simulink model "TURBINE"  (R2016a)
settings: Solver=VariableStepAuto  StartTime=0.0  StopTime=10.0  RelTol=1e-3
values from neighbouring files (symbols this model uses):
  C_l0 = 1.2195    [zmienne.m]
  COF = 3.0326    [zmienne.m]
  CP_fw = 1.218    [zmienne.m]
  ETA_hp = 0.861    [zmienne.m]
  ETA_lp = 0.861    [zmienne.m]
  G_1t = 1.65    [zmienne.m]
  G_vt = 1.5    [zmienne.m]
  H_4p = 958.4    [zmienne.m]
  H_et = 22.589    [zmienne.m]
  HE_fw2 = 863.76    [zmienne.m]
  I_t = 199642    [zmienne.m]
  J = 5.4027    [Pressurizer_constants.m]    (also in zmienne.m = 5.404)
  K10 = 0.53    [zmienne.m]
  K11 = -0.45    [zmienne.m]
  K12 = 0.1    [zmienne.m]
  K13 = -0.017    [zmienne.m]
  K14 = 0.14    [zmienne.m]
  K15 = 0.85612    [zmienne.m]
  K_1c = 1.27453    [zmienne.m]
  K_1co = 37.74    [zmienne.m]
  K_2c = 1068.8    [zmienne.m]
  K_2co = 32    [zmienne.m]
  K_3co = 1092.8    [zmienne.m]
  K_3t = 431.435    [zmienne.m]
  K_4co = 13    [zmienne.m]
  K_5co = 1054    [zmienne.m]
  K_6co = -18    [zmienne.m]
  K_7co = 0.8833    [zmienne.m]
  K_8co = 0.0166    [zmienne.m]
  K_bhp = 0.1634    [zmienne.m]
  K_blp = 0.2174    [zmienne.m]
  KT_t = 1.414    [zmienne.m]
  ML_co = 41422.9    [zmienne.m]
  N_t0 = 60    [zmienne.m]
  P_co = 1    [zmienne.m]
  P_ct = 790    [zmienne.m]
  P_rt = 160    [zmienne.m]
  PI = 3.141    [zmienne.m]
  tau_1t = 4    [zmienne.m]
  tau_2p = 10    [zmienne.m]
  tau_co = 7    [zmienne.m]
  tau_h1 = 65    [zmienne.m]
  tau_h2 = 22    [zmienne.m]
  tau_r1 = 3    [zmienne.m]
  tau_r2 = 10    [zmienne.m]
  tau_w2 = 2    [zmienne.m]
  tau_w3 = 10    [zmienne.m]
  V_ct = 200    [zmienne.m]
  V_ft = 0.018152    [zmienne.m]
  V_rt = 20000    [zmienne.m]
  W_fw = 1036.39    [zmienne.m]
  W_nt = 9.75    [zmienne.m]
  X10 = 931.8    [zmienne.m]
  X11 = 1180    [zmienne.m]
  X12 = 5.556    [zmienne.m]
  X13 = 402.94    [zmienne.m]
  X9 = 251.31    [zmienne.m]
  Z_t = 0.67    [zmienne.m]
undefined symbols (not defined in the file or in its folder): magnitude
settings Model: Creator=Użytkownik  LastModifiedBy=Użytkownik
settings GRTTargetCC: GeneratePreprocessorConditionals=Use local settings

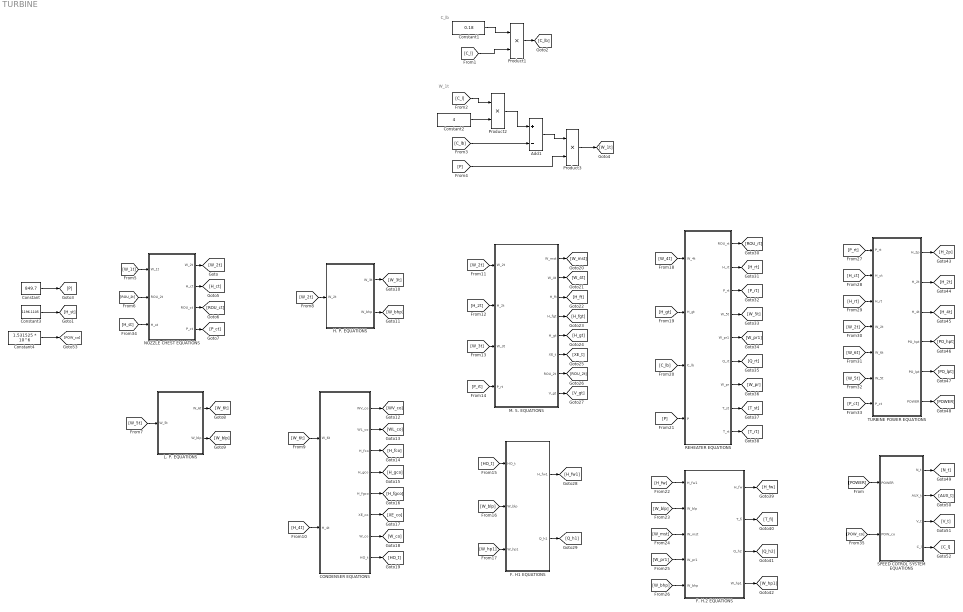
== system TURBINE ==
  note: W_1t
  note: C_lb
  Add1 : Sum  Inputs=+-
  CONDENSER EQUATIONS : Subsystem
  Constant : Constant  Value=849.7
  Constant1 : Constant  Value=0.18
  Constant2 : Constant  Value=4
  Constant3 : Constant  Value=1196.1105
  Constant4 : Constant  Value=1.531525 * 10^6
  "F. H.2 EQUATIONS " : Subsystem
  F. H1 EQUATIONS : Subsystem
  H. P. EQUATIONS : Subsystem
  L. P. EQUATIONS : Subsystem
  M. S. EQUATIONS : Subsystem
  NOZZLE CHEST EQUATIONS : Subsystem
  Product1 : Product
  Product2 : Product
  Product3 : Product
  REHEATER EQUATIONS : Subsystem
  SPEED COTROL SYSTEM EQUATIONS : Subsystem
  TURBINE POWER EQUATIONS : Subsystem
  wires:
  Constant1/1 -> Product1/1
  [C_l] -> Product1/2
  Product1/1 -> [C_lb]
  [C_l] -> Product2/1
  Constant2/1 -> Product2/2
  [C_lb] -> Add1/2
  Product2/1 -> Add1/1
  Add1/1 -> Product3/1
  [P] -> Product3/2
  Product3/1 -> [W_1t]
  NOZZLE CHEST EQUATIONS/1(W_2t) -> [W_2t]
  NOZZLE CHEST EQUATIONS/2(H_ct) -> [H_ct]
  NOZZLE CHEST EQUATIONS/3(ROU_ct) -> [ROU_ct]
  NOZZLE CHEST EQUATIONS/4(P_ct) -> [P_ct]
  L. P. EQUATIONS/1(W_6t) -> [W_6t]
  L. P. EQUATIONS/2(W_blp) -> [W_blp]
  H. P. EQUATIONS/1(W_3t) -> [W_3t]
  H. P. EQUATIONS/2(W_bhp) -> [W_bhp]
  CONDENSER EQUATIONS/1(WV_co) -> [WV_co]
  CONDENSER EQUATIONS/2(WL_co) -> [WL_co]
  CONDENSER EQUATIONS/3(H_fco) -> [H_fco]
  CONDENSER EQUATIONS/4(H_gco) -> [H_gco]
  CONDENSER EQUATIONS/5(H_fgco) -> [H_fgco]
  CONDENSER EQUATIONS/6(XE_co) -> [XE_co]
  CONDENSER EQUATIONS/7(W_co) -> [W_co]
  CONDENSER EQUATIONS/8(HO_t) -> [HO_t]
  M. S. EQUATIONS/1(W_mst) -> [W_mst]
  M. S. EQUATIONS/2(W_4t) -> [W_4t]
  M. S. EQUATIONS/3(H_ft) -> [H_ft]
  M. S. EQUATIONS/4(H_fgt) -> [H_fgt]
  M. S. EQUATIONS/5(H_gt) -> [H_gt]
  M. S. EQUATIONS/6(XE_t) -> [XE_t]
  M. S. EQUATIONS/7(ROU_2t) -> [ROU_2t]
  M. S. EQUATIONS/8(V_gt) -> [V_gt]
  F. H1 EQUATIONS/1(H_fw1) -> [H_fw1]
  F. H1 EQUATIONS/2(Q_h1) -> [Q_h1]
  REHEATER EQUATIONS/1("ROU_rt ") -> [ROU_rt]
  REHEATER EQUATIONS/2(H_rt) -> [H_rt]
  REHEATER EQUATIONS/3(P_rt) -> [P_rt]
  REHEATER EQUATIONS/4(W_5t) -> [W_5t]
  REHEATER EQUATIONS/5(W_pr1) -> [W_pr1]
  REHEATER EQUATIONS/6(Q_rt) -> [Q_rt]
  REHEATER EQUATIONS/7(W_pr) -> [W_pr]
  REHEATER EQUATIONS/8(T_st) -> [T_st]
  REHEATER EQUATIONS/9(T_rt) -> [T_rt]
  "F. H.2 EQUATIONS "/1(H_fw) -> [H_fw]
  "F. H.2 EQUATIONS "/2(T_fi) -> [T_fi]
  "F. H.2 EQUATIONS "/3(Q_h2) -> [Q_h2]
  "F. H.2 EQUATIONS "/4(W_hp1) -> [W_hp1]
  TURBINE POWER EQUATIONS/1(H_2p) -> [H_2p]
  TURBINE POWER EQUATIONS/2(H_2t) -> [H_2t]
  TURBINE POWER EQUATIONS/3(H_4t) -> [H_4t]
  TURBINE POWER EQUATIONS/4(PO_hpt) -> [PO_hpt]
  TURBINE POWER EQUATIONS/5(PO_lpt) -> [PO_lpt]
  TURBINE POWER EQUATIONS/6(POWER) -> [POWER]
  SPEED COTROL SYSTEM EQUATIONS/1(N_t) -> [N_t]
  SPEED COTROL SYSTEM EQUATIONS/2(AUX_t) -> [AUX_t]
  SPEED COTROL SYSTEM EQUATIONS/3(V_t) -> [V_t]
  SPEED COTROL SYSTEM EQUATIONS/4(C_l) -> [C_l]
  [W_1t] -> NOZZLE CHEST EQUATIONS/1(W_1t)
  [ROU_2t] -> NOZZLE CHEST EQUATIONS/2(ROU_2t)
  [W_5t] -> L. P. EQUATIONS/1(W_5t)
  [W_2t] -> H. P. EQUATIONS/1(W_2t)
  [W_6t] -> CONDENSER EQUATIONS/1(W_6t)
  [H_4t] -> CONDENSER EQUATIONS/2(H_4t)
  [W_2t] -> M. S. EQUATIONS/1(W_2t)
  [H_2t] -> M. S. EQUATIONS/2(H_2t)
  [W_3t] -> M. S. EQUATIONS/3(W_3t)
  [P_rt] -> M. S. EQUATIONS/4(P_rt)
  [HO_t] -> F. H1 EQUATIONS/1(HO_t)
  [W_blp] -> F. H1 EQUATIONS/2(W_blp)
  [W_hp1] -> F. H1 EQUATIONS/3(W_hp1)
  [W_4t] -> REHEATER EQUATIONS/1(W_4t)
  [H_gt] -> REHEATER EQUATIONS/2(H_gt)
  [C_lb] -> REHEATER EQUATIONS/3(C_lb)
  [P] -> REHEATER EQUATIONS/4(P)
  [H_fw] -> "F. H.2 EQUATIONS "/1(H_fw1)
  [W_blp] -> "F. H.2 EQUATIONS "/2(W_blp)
  [W_mst] -> "F. H.2 EQUATIONS "/3(W_mst)
  [W_pr1] -> "F. H.2 EQUATIONS "/4(W_pr1)
  [W_bhp] -> "F. H.2 EQUATIONS "/5(W_bhp)
  [P_rt] -> TURBINE POWER EQUATIONS/1(P_rt)
  [H_ct] -> TURBINE POWER EQUATIONS/2(H_ct)
  [H_rt] -> TURBINE POWER EQUATIONS/3(H_rt)
  [W_2t] -> TURBINE POWER EQUATIONS/4(W_2t)
  [W_6t] -> TURBINE POWER EQUATIONS/5(W_6t)
  [W_5t] -> TURBINE POWER EQUATIONS/6(W_5t)
  [P_ct] -> TURBINE POWER EQUATIONS/7(P_ct)
  [POWER] -> SPEED COTROL SYSTEM EQUATIONS/1(POWER)
  Constant/1 -> [P]
  Constant3/1 -> [H_st]
  Constant4/1 -> [POW_co]
  [H_st] -> NOZZLE CHEST EQUATIONS/3(H_st)
  [POW_co] -> SPEED COTROL SYSTEM EQUATIONS/2(POW_co)

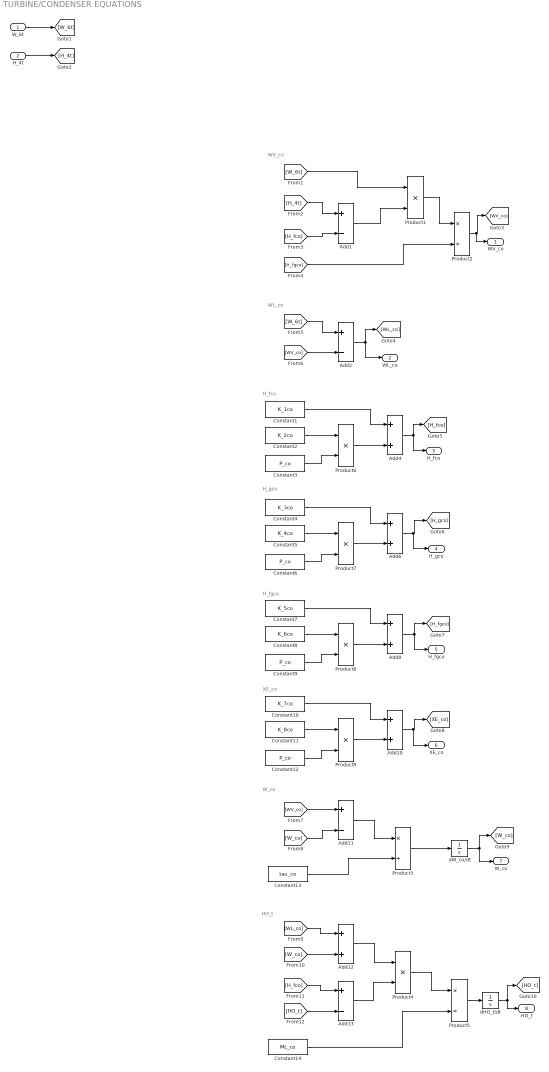
== system TURBINE/CONDENSER EQUATIONS ==
  note: HO_t
  note: W_co
  note: XE_co
  note: H_fgco
  note: H_gco
  note: H_fco
  note: WL_co
  note: WV_co
  W_6t : Inport
  H_4t : Inport  Port=2
  Add{1..2,11,13} (4 alike) : Sum  Inputs=+-
  Add{4,6,8,10,12} (5 alike) : Sum
  Constant1 : Constant  Value=K_1co
  Constant10 : Constant  Value=K_7co
  Constant11 : Constant  Value=K_8co
  Constant{3,6,9,12} (4 alike) : Constant  Value=P_co
  Constant13 : Constant  Value=tau_co
  Constant14 : Constant  Value=ML_co
  Constant2 : Constant  Value=K_2co
  Constant4 : Constant  Value=K_3co
  Constant5 : Constant  Value=K_4co
  Constant7 : Constant  Value=K_5co
  Constant8 : Constant  Value=K_6co
  Product{1,4,6..9} (6 alike) : Product
  Product2 : Product  Inputs=*/
  Product3 : Product  Inputs=*/
  Product5 : Product  Inputs=*/
  dHO_t/dt : Integrator  InitialCondition=69.713
  dW_co/dt : Integrator  InitialCondition=2072.5
  WV_co : Outport
  WL_co : Outport  Port=2
  H_fco : Outport  Port=3
  H_gco : Outport  Port=4
  H_fgco : Outport  Port=5
  XE_co : Outport  Port=6
  W_co : Outport  Port=7
  HO_t : Outport  Port=8
  wires:
  W_6t/1 -> [W_6t]
  H_4t/1 -> [H_4t]
  [H_4t] -> Add1/1
  [H_fco] -> Add1/2
  [W_6t] -> Product1/1
  Add1/1 -> Product1/2
  Product1/1 -> Product2/1
  [H_fgco] -> Product2/2
  Product2/1 -> WV_co/1, [WV_co]
  [W_6t] -> Add2/1
  [WV_co] -> Add2/2
  Add2/1 -> [WL_co], WL_co/1
  Constant2/1 -> Product6/1
  Constant3/1 -> Product6/2
  Constant1/1 -> Add4/1
  Constant5/1 -> Product7/1
  Constant6/1 -> Product7/2
  Constant4/1 -> Add6/1
  Product7/1 -> Add6/2
  Constant8/1 -> Product8/1
  Constant9/1 -> Product8/2
  Constant7/1 -> Add8/1
  Product8/1 -> Add8/2
  Constant11/1 -> Product9/1
  Constant12/1 -> Product9/2
  Constant10/1 -> Add10/1
  Product9/1 -> Add10/2
  Add4/1 -> H_fco/1, [H_fco]
  Add6/1 -> H_gco/1, [H_gco]
  Add8/1 -> [H_fgco], H_fgco/1
  Add10/1 -> XE_co/1, [XE_co]
  [WV_co] -> Add11/1
  [W_co] -> Add11/2
  Add11/1 -> Product3/1
  Constant13/1 -> Product3/2
  Product3/1 -> dW_co/dt/1
  dW_co/dt/1 -> W_co/1, [W_co]
  [W_co] -> Add12/2
  [WL_co] -> Add12/1
  [H_fco] -> Add13/1
  [HO_t] -> Add13/2
  Add12/1 -> Product4/1
  Add13/1 -> Product4/2
  Product4/1 -> Product5/1
  Constant14/1 -> Product5/2
  Product5/1 -> dHO_t/dt/1
  dHO_t/dt/1 -> HO_t/1, [HO_t]
  Product6/1 -> Add4/2

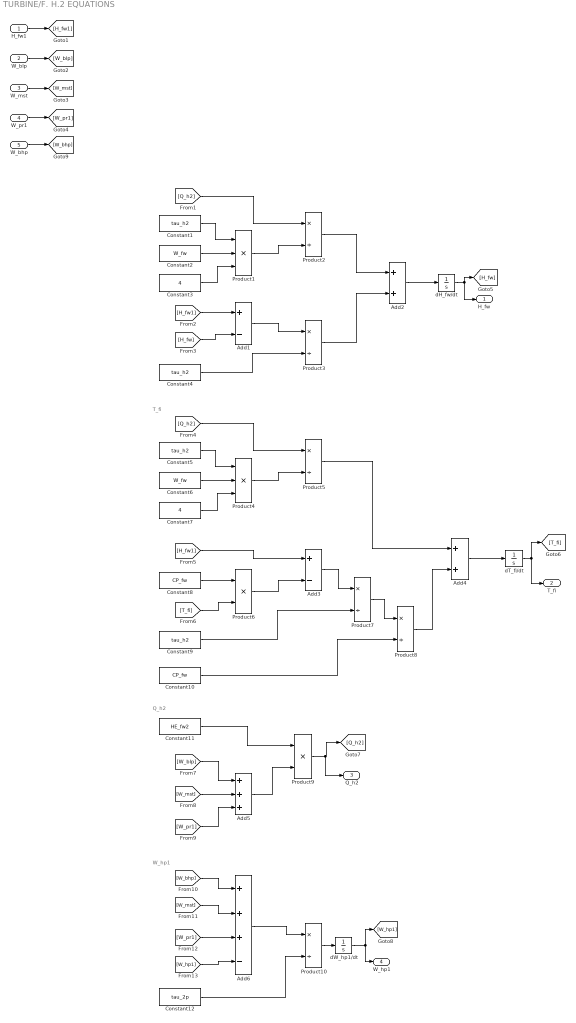
== system TURBINE/F. H.2 EQUATIONS  ==
  note: W_hp1
  note: Q_h2
  note: T_fi
  H_fw1 : Inport
  W_blp : Inport  Port=2
  W_mst : Inport  Port=3
  W_pr1 : Inport  Port=4
  W_bhp : Inport  Port=5
  Add1 : Sum  Inputs=+-
  Add2 : Sum
  Add3 : Sum  Inputs=+-
  Add4 : Sum
  Add5 : Sum  Inputs=3
  Add6 : Sum  Inputs=+++-
  Constant{1,4..5,9} (4 alike) : Constant  Value=tau_h2
  Constant10 : Constant  Value=CP_fw
  Constant11 : Constant  Value=HE_fw2
  Constant12 : Constant  Value=tau_2p
  Constant2 : Constant  Value=W_fw
  Constant3 : Constant  Value=4
  Constant6 : Constant  Value=W_fw
  Constant7 : Constant  Value=4
  Constant8 : Constant  Value=CP_fw
  Product1 : Product  Inputs=3
  Product{2..3,5,7..8,10} (6 alike) : Product  Inputs=*/
  Product4 : Product  Inputs=3
  Product6 : Product
  Product9 : Product
  dH_fw/dt : Integrator  InitialCondition=529.15
  dT_fi/dt : Integrator  InitialCondition=434.3
  dW_hp1/dt : Integrator  InitialCondition=1217.8
  H_fw : Outport
  T_fi : Outport  Port=2
  Q_h2 : Outport  Port=3
  W_hp1 : Outport  Port=4
  wires:
  H_fw1/1 -> [H_fw1]
  W_blp/1 -> [W_blp]
  W_mst/1 -> [W_mst]
  W_pr1/1 -> [W_pr1]
  Constant1/1 -> Product1/1
  Constant2/1 -> Product1/2
  Constant3/1 -> Product1/3
  [Q_h2] -> Product2/1
  Product1/1 -> Product2/2
  [H_fw1] -> Add1/1
  [H_fw] -> Add1/2
  Add1/1 -> Product3/1
  Constant4/1 -> Product3/2
  Product2/1 -> Add2/1
  Product3/1 -> Add2/2
  Add2/1 -> dH_fw/dt/1
  dH_fw/dt/1 -> H_fw/1, [H_fw]
  Constant5/1 -> Product4/1
  Constant6/1 -> Product4/2
  Constant7/1 -> Product4/3
  [Q_h2] -> Product5/1
  Product4/1 -> Product5/2
  Constant8/1 -> Product6/1
  [T_fi] -> Product6/2
  [H_fw1] -> Add3/1
  Product6/1 -> Add3/2
  Add3/1 -> Product7/1
  Constant9/1 -> Product7/2
  Product5/1 -> Add4/1
  [W_blp] -> Add5/1
  [W_mst] -> Add5/2
  [W_pr1] -> Add5/3
  Constant11/1 -> Product9/1
  Add5/1 -> Product9/2
  dT_fi/dt/1 -> T_fi/1, [T_fi]
  Product9/1 -> Q_h2/1, [Q_h2]
  W_bhp/1 -> [W_bhp]
  [W_bhp] -> Add6/1
  [W_mst] -> Add6/2
  [W_pr1] -> Add6/3
  [W_hp1] -> Add6/4
  Add6/1 -> Product10/1
  Constant12/1 -> Product10/2
  Product10/1 -> dW_hp1/dt/1
  dW_hp1/dt/1 -> W_hp1/1, [W_hp1]
  Add4/1 -> dT_fi/dt/1
  Constant10/1 -> Product8/2
  Product7/1 -> Product8/1
  Product8/1 -> Add4/2

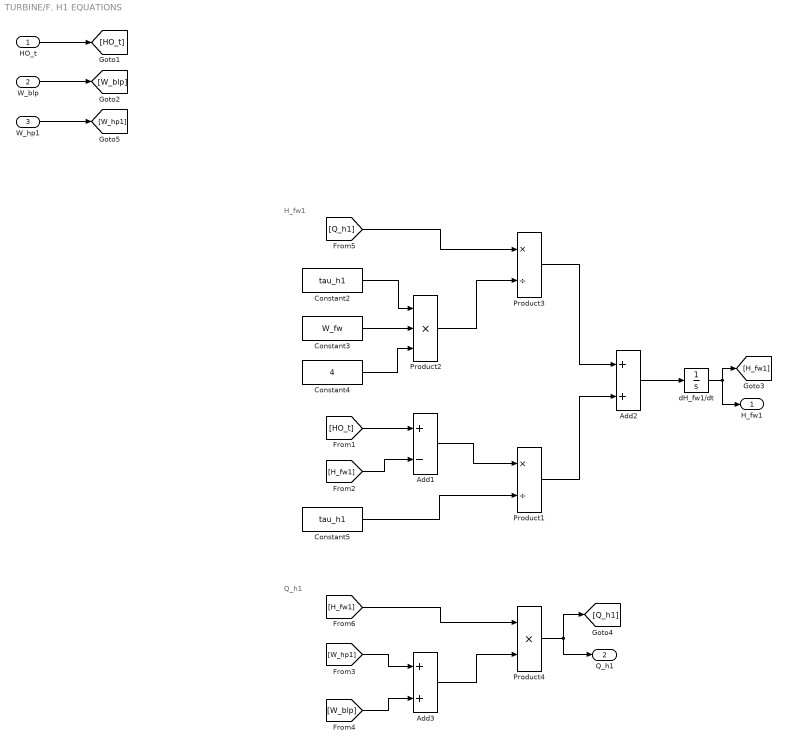
== system TURBINE/F. H1 EQUATIONS ==
  note: Q_h1
  note: H_fw1
  HO_t : Inport
  W_blp : Inport  Port=2
  W_hp1 : Inport  Port=3
  Add1 : Sum  Inputs=+-
  Add2 : Sum
  Add3 : Sum
  Constant2 : Constant  Value=tau_h1
  Constant3 : Constant  Value=W_fw
  Constant4 : Constant  Value=4
  Constant5 : Constant  Value=tau_h1
  Product1 : Product  Inputs=*/
  Product2 : Product  Inputs=***
  Product3 : Product  Inputs=*/
  Product4 : Product
  dH_fw1/dt : Integrator  InitialCondition=280.4
  H_fw1 : Outport
  Q_h1 : Outport  Port=2
  wires:
  HO_t/1 -> [HO_t]
  W_blp/1 -> [W_blp]
  [HO_t] -> Add1/1
  [H_fw1] -> Add1/2
  Add1/1 -> Product1/1
  Constant5/1 -> Product1/2
  Constant2/1 -> Product2/1
  Constant3/1 -> Product2/2
  Constant4/1 -> Product2/3
  Product2/1 -> Product3/2
  [Q_h1] -> Product3/1
  Product3/1 -> Add2/1
  Product1/1 -> Add2/2
  Add2/1 -> dH_fw1/dt/1
  dH_fw1/dt/1 -> [H_fw1], H_fw1/1
  [W_hp1] -> Add3/1
  [W_blp] -> Add3/2
  [H_fw1] -> Product4/1
  Add3/1 -> Product4/2
  Product4/1 -> Q_h1/1, [Q_h1]
  W_hp1/1 -> [W_hp1]

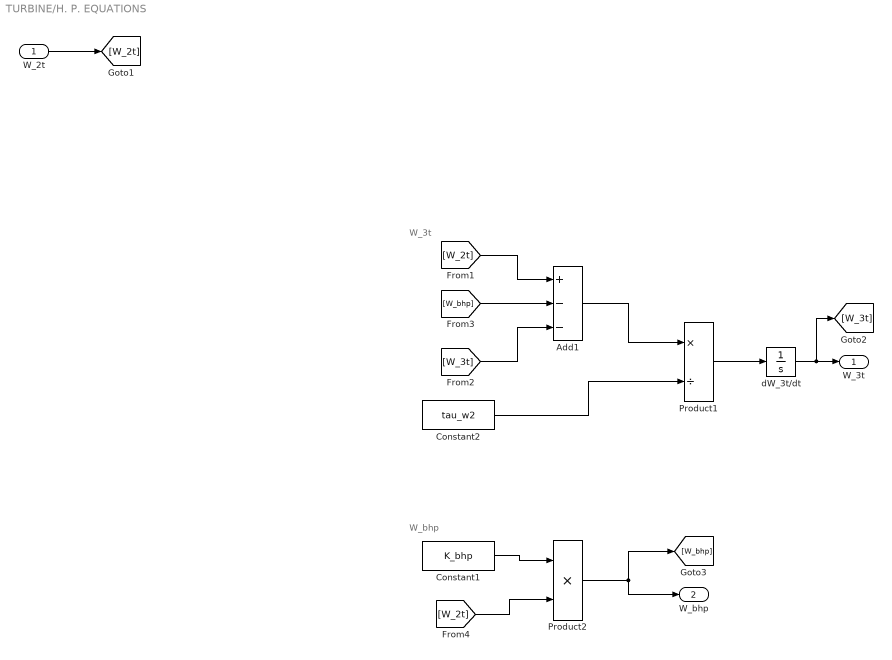
== system TURBINE/H. P. EQUATIONS ==
  note: W_bhp
  note: W_3t
  W_2t : Inport
  Add1 : Sum  Inputs=+--
  Constant1 : Constant  Value=K_bhp
  Constant2 : Constant  Value=tau_w2
  Product1 : Product  Inputs=*/
  Product2 : Product
  dW_3t/dt : Integrator  InitialCondition=3311.56
  W_3t : Outport
  W_bhp : Outport  Port=2
  wires:
  W_2t/1 -> [W_2t]
  [W_2t] -> Add1/1
  [W_bhp] -> Add1/2
  [W_3t] -> Add1/3
  Add1/1 -> Product1/1
  Constant2/1 -> Product1/2
  Product1/1 -> dW_3t/dt/1
  dW_3t/dt/1 -> [W_3t], W_3t/1
  Constant1/1 -> Product2/1
  [W_2t] -> Product2/2
  Product2/1 -> [W_bhp], W_bhp/1

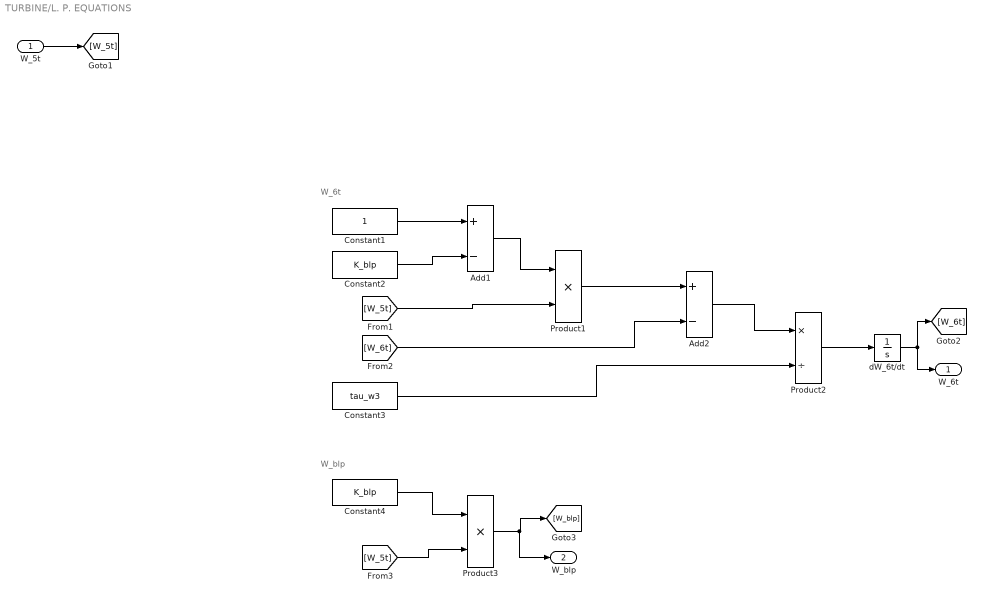
== system TURBINE/L. P. EQUATIONS ==
  note: W_blp
  note: W_6t
  W_5t : Inport
  Add1 : Sum  Inputs=+-
  Add2 : Sum  Inputs=+-
  Constant1 : Constant
  Constant2 : Constant  Value=K_blp
  Constant3 : Constant  Value=tau_w3
  Constant4 : Constant  Value=K_blp
  Product1 : Product
  Product2 : Product  Inputs=*/
  Product3 : Product
  dW_6t/dt : Integrator  InitialCondition=2303
  W_6t : Outport
  W_blp : Outport  Port=2
  wires:
  W_5t/1 -> [W_5t]
  Constant1/1 -> Add1/1
  Constant2/1 -> Add1/2
  Add1/1 -> Product1/1
  [W_5t] -> Product1/2
  Product1/1 -> Add2/1
  [W_6t] -> Add2/2
  Add2/1 -> Product2/1
  Constant3/1 -> Product2/2
  Product2/1 -> dW_6t/dt/1
  dW_6t/dt/1 -> [W_6t], W_6t/1
  Constant4/1 -> Product3/1
  [W_5t] -> Product3/2
  Product3/1 -> W_blp/1, [W_blp]

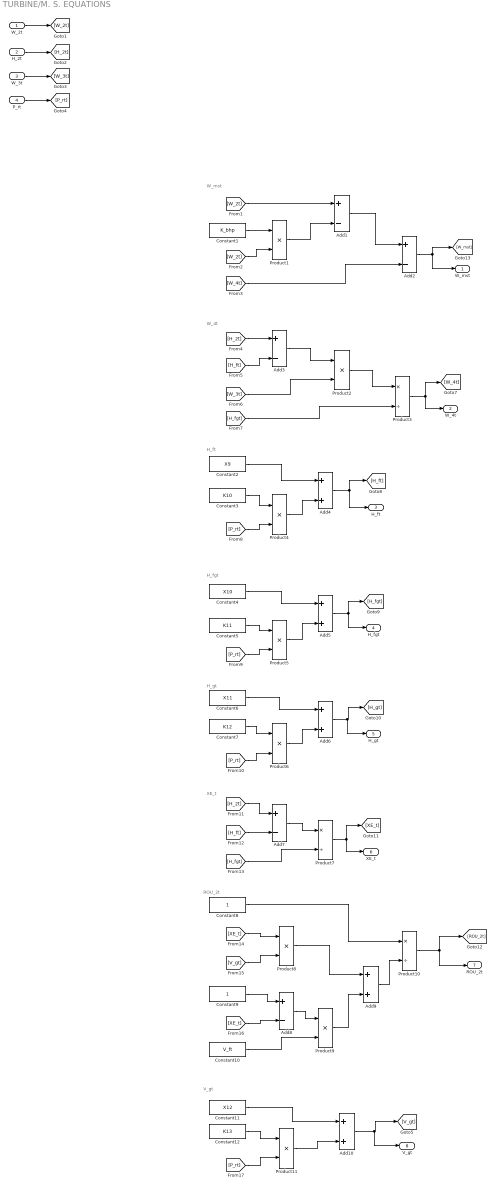
== system TURBINE/M. S. EQUATIONS ==
  note: V_gt
  note: ROU_2t
  note: XE_t
  note: H_gt
  note: H_fgt
  note: H_ft
  note: W_4t
  note: W_mst
  W_2t : Inport
  H_2t : Inport  Port=2
  W_3t : Inport  Port=3
  P_rt : Inport  Port=4
  Add{1..3,7..8} (5 alike) : Sum  Inputs=+-
  Add{4..6,9..10} (5 alike) : Sum
  Constant1 : Constant  Value=K_bhp
  Constant10 : Constant  Value=V_ft
  Constant11 : Constant  Value=X12
  Constant12 : Constant  Value=K13
  Constant2 : Constant  Value=X9
  Constant3 : Constant  Value=K10
  Constant4 : Constant  Value=X10
  Constant5 : Constant  Value=K11
  Constant6 : Constant  Value=X11
  Constant7 : Constant  Value=K12
  Constant8 : Constant
  Constant9 : Constant
  Product{1..2,4..6,8..9,11} (8 alike) : Product
  Product10 : Product  Inputs=*/
  Product3 : Product  Inputs=*/
  Product7 : Product  Inputs=*/
  W_mst : Outport
  W_4t : Outport  Port=2
  H_ft : Outport  Port=3
  H_fgt : Outport  Port=4
  H_gt : Outport  Port=5
  XE_t : Outport  Port=6
  ROU_2t : Outport  Port=7
  V_gt : Outport  Port=8
  wires:
  W_2t/1 -> [W_2t]
  H_2t/1 -> [H_2t]
  W_3t/1 -> [W_3t]
  P_rt/1 -> [P_rt]
  Constant1/1 -> Product1/1
  [W_2t] -> Product1/2
  [W_2t] -> Add1/1
  Product1/1 -> Add1/2
  Add1/1 -> Add2/1
  [W_4t] -> Add2/2
  Add2/1 -> W_mst/1, [W_mst]
  [H_2t] -> Add3/1
  [H_ft] -> Add3/2
  Add3/1 -> Product2/1
  [W_3t] -> Product2/2
  Product2/1 -> Product3/1
  [H_fgt] -> Product3/2
  Product3/1 -> W_4t/1, [W_4t]
  Constant3/1 -> Product4/1
  [P_rt] -> Product4/2
  Constant2/1 -> Add4/1
  Product4/1 -> Add4/2
  Add4/1 -> H_ft/1, [H_ft]
  Constant5/1 -> Product5/1
  [P_rt] -> Product5/2
  Constant4/1 -> Add5/1
  Product5/1 -> Add5/2
  Add5/1 -> H_fgt/1, [H_fgt]
  Constant7/1 -> Product6/1
  [P_rt] -> Product6/2
  Constant6/1 -> Add6/1
  Product6/1 -> Add6/2
  Add6/1 -> H_gt/1, [H_gt]
  [H_2t] -> Add7/1
  [H_ft] -> Add7/2
  Add7/1 -> Product7/1
  [H_fgt] -> Product7/2
  Product7/1 -> XE_t/1, [XE_t]
  [XE_t] -> Product8/1
  [V_gt] -> Product8/2
  Constant9/1 -> Add8/1
  [XE_t] -> Add8/2
  Add8/1 -> Product9/1
  Constant10/1 -> Product9/2
  Product8/1 -> Add9/1
  Product9/1 -> Add9/2
  Constant8/1 -> Product10/1
  Add9/1 -> Product10/2
  Product10/1 -> ROU_2t/1, [ROU_2t]
  Constant12/1 -> Product11/1
  [P_rt] -> Product11/2
  Constant11/1 -> Add10/1
  Product11/1 -> Add10/2
  Add10/1 -> V_gt/1, [V_gt]

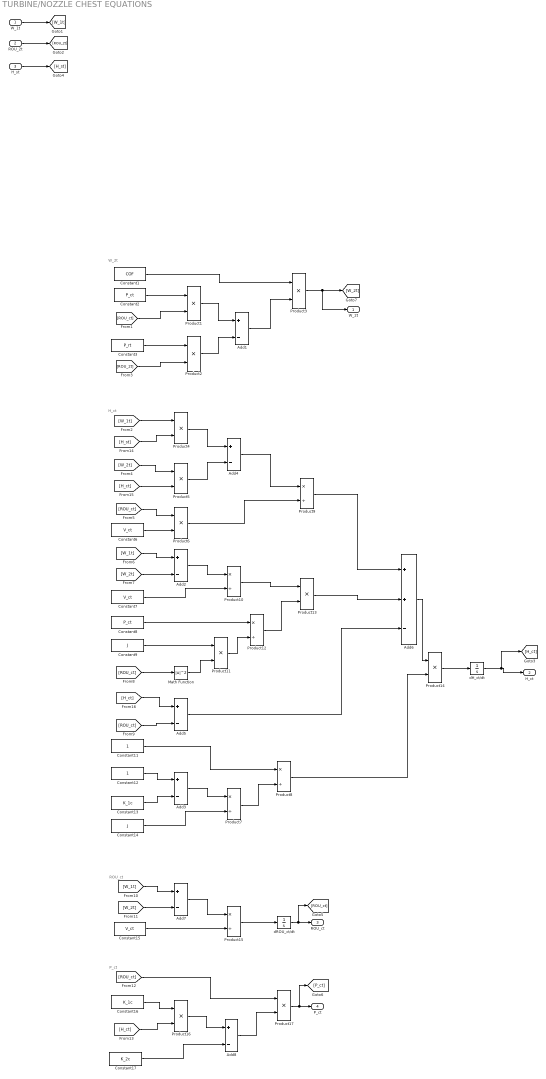
== system TURBINE/NOZZLE CHEST EQUATIONS ==
  note: P_ct
  note: ROU_ct
  note: H_ct
  note: W_2t
  W_1t : Inport
  ROU_2t : Inport  Port=2
  H_st : Inport  Port=3
  Add{1..5,7..8} (7 alike) : Sum  Inputs=+-
  Add6 : Sum  Inputs=++-
  Constant1 : Constant  Value=COF
  Constant11 : Constant
  Constant12 : Constant
  Constant13 : Constant  Value=K_1c
  Constant14 : Constant  Value=J
  Constant15 : Constant  Value=V_ct
  Constant16 : Constant  Value=K_1c
  Constant17 : Constant  Value=K_2c
  Constant2 : Constant  Value=P_ct
  Constant3 : Constant  Value=P_rt
  Constant6 : Constant  Value=V_ct
  Constant7 : Constant  Value=V_ct
  Constant8 : Constant  Value=P_ct
  Constant9 : Constant  Value=J
  Math Function : Math  Operator=magnitude^2  SaturateOnIntegerOverflow=on
  Product{1..6,11,13..14,16..17} (11 alike) : Product
  Product{7..10,12,15} (6 alike) : Product  Inputs=*/
  dH_ct/dt : Integrator  InitialCondition=1196.1
  dROU_ct/dt : Integrator  InitialCondition=1.7337
  W_2t : Outport
  H_ct : Outport  Port=2
  ROU_ct : Outport  Port=3
  P_ct : Outport  Port=4
  wires:
  W_1t/1 -> [W_1t]
  ROU_2t/1 -> [ROU_2t]
  Constant3/1 -> Product2/1
  [ROU_2t] -> Product2/2
  Constant2/1 -> Product1/1
  [ROU_ct] -> Product1/2
  Product1/1 -> Add1/1
  Product2/1 -> Add1/2
  Constant1/1 -> Product3/1
  Add1/1 -> Product3/2
  Product3/1 -> W_2t/1, [W_2t]
  [W_1t] -> Product4/1
  [H_st] -> Product4/2
  [W_2t] -> Product5/1
  [H_ct] -> Product5/2
  [ROU_ct] -> Product6/1
  Constant6/1 -> Product6/2
  [W_1t] -> Add2/1
  [W_2t] -> Add2/2
  [ROU_ct] -> Math Function/1
  Constant12/1 -> Add3/1
  Constant13/1 -> Add3/2
  Add3/1 -> Product7/1
  Constant14/1 -> Product7/2
  Constant11/1 -> Product8/1
  Product7/1 -> Product8/2
  Product4/1 -> Add4/1
  Product5/1 -> Add4/2
  Add4/1 -> Product9/1
  Product6/1 -> Product9/2
  Add2/1 -> Product10/1
  Constant7/1 -> Product10/2
  Constant9/1 -> Product11/1
  Math Function/1 -> Product11/2
  Constant8/1 -> Product12/1
  Product11/1 -> Product12/2
  Product10/1 -> Product13/1
  Product12/1 -> Product13/2
  [H_ct] -> Add5/1
  [ROU_ct] -> Add5/2
  Product9/1 -> Add6/1
  Product13/1 -> Add6/2
  Add5/1 -> Add6/3
  Add6/1 -> Product14/1
  Product8/1 -> Product14/2
  Product14/1 -> dH_ct/dt/1
  dH_ct/dt/1 -> [H_ct], H_ct/1
  [W_2t] -> Add7/2
  [W_1t] -> Add7/1
  Add7/1 -> Product15/1
  Constant15/1 -> Product15/2
  Product15/1 -> dROU_ct/dt/1
  dROU_ct/dt/1 -> [ROU_ct], ROU_ct/1
  Constant16/1 -> Product16/1
  [H_ct] -> Product16/2
  Product16/1 -> Add8/1
  Constant17/1 -> Add8/2
  [ROU_ct] -> Product17/1
  Add8/1 -> Product17/2
  Product17/1 -> [P_ct], P_ct/1
  H_st/1 -> [H_st]

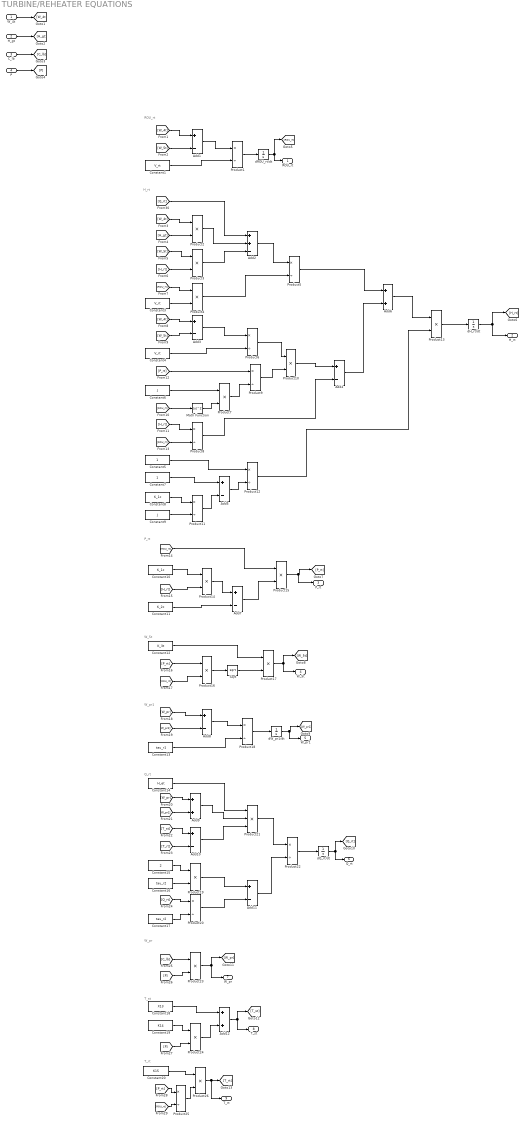
== system TURBINE/REHEATER EQUATIONS ==
  note: T_rt
  note: T_st
  note: W_pr
  note: Q_rt
  note: W_pr1
  note: W_5t
  note: P_rt
  note: H_rt
  note: ROU_rt
  W_4t : Inport
  H_gt : Inport  Port=2
  C_lb : Inport  Port=3
  P : Inport  Port=4
  Add{1,3..5,7..8,10..11} (8 alike) : Sum  Inputs=+-
  Add12 : Sum
  Add2 : Sum  Inputs=++-
  Add6 : Sum
  Add9 : Sum
  Constant1 : Constant  Value=V_rt
  Constant10 : Constant  Value=K_1c
  Constant11 : Constant  Value=K_2c
  Constant12 : Constant  Value=K_3t
  Constant13 : Constant  Value=tau_r1
  Constant14 : Constant  Value=H_et
  Constant15 : Constant  Value=2
  Constant16 : Constant  Value=tau_r2
  Constant17 : Constant  Value=tau_r2
  Constant18 : Constant  Value=X13
  Constant19 : Constant  Value=K14
  Constant20 : Constant  Value=K15
  Constant3 : Constant  Value=V_rt
  Constant4 : Constant  Value=V_rt
  Constant5 : Constant
  Constant6 : Constant  Value=J
  Constant7 : Constant
  Constant8 : Constant  Value=K_1c
  Constant9 : Constant  Value=J
  Math Function : Math  Operator=magnitude^2  SaturateOnIntegerOverflow=on
  Product{1,5..6,8..9,11..12,18,20,22,25} (11 alike) : Product  Inputs=*/
  Product{2..4,7,10,13..17,19,23..24,26} (14 alike) : Product
  Product21 : Product  Inputs=3
  Sqrt : Sqrt  SaturateOnIntegerOverflow=on
  dH_rt/dt : Integrator  InitialCondition=1269.7
  dQ_rt/dt : Integrator  InitialCondition=216931
  dROU_rt/dt : Integrator  InitialCondition=0.291
  dW_pr1/dt : Integrator  InitialCondition=186.36
  "ROU_rt " : Outport
  H_rt : Outport  Port=2
  P_rt : Outport  Port=3
  W_5t : Outport  Port=4
  W_pr1 : Outport  Port=5
  Q_rt : Outport  Port=6
  W_pr : Outport  Port=7
  T_st : Outport  Port=8
  T_rt : Outport  Port=9
  wires:
  W_4t/1 -> [W_4t]
  H_gt/1 -> [H_gt]
  C_lb/1 -> [C_lb]
  P/1 -> [P]
  [W_5t] -> Add1/2
  [W_4t] -> Add1/1
  Add1/1 -> Product1/1
  Constant1/1 -> Product1/2
  Product1/1 -> dROU_rt/dt/1
  dROU_rt/dt/1 -> "ROU_rt "/1, [ROU_rt]
  [H_gt] -> Product2/2
  [W_4t] -> Product2/1
  [H_rt] -> Product3/2
  [W_5t] -> Product3/1
  Constant3/1 -> Product4/2
  [ROU_rt] -> Product4/1
  [Q_rt] -> Add2/1
  Product2/1 -> Add2/2
  Product3/1 -> Add2/3
  Add2/1 -> Product5/1
  Product4/1 -> Product5/2
  [W_4t] -> Add3/1
  [W_5t] -> Add3/2
  Add3/1 -> Product6/1
  Constant4/1 -> Product6/2
  [ROU_rt] -> Math Function/1
  Constant6/1 -> Product7/1
  Math Function/1 -> Product7/2
  [ROU_rt] -> Product8/2
  [H_rt] -> Product8/1
  Product8/1 -> Add4/2
  [P_rt] -> Product9/1
  Product6/1 -> Product10/1
  Constant9/1 -> Product11/2
  Constant8/1 -> Product11/1
  Constant7/1 -> Add5/1
  Product11/1 -> Add5/2
  Constant5/1 -> Product12/1
  Add5/1 -> Product12/2
  Product12/1 -> Product13/2
  Product5/1 -> Add6/1
  dH_rt/dt/1 -> H_rt/1, [H_rt]
  Constant10/1 -> Product14/1
  [H_rt] -> Product14/2
  Product14/1 -> Add7/1
  Constant11/1 -> Add7/2
  [ROU_rt] -> Product15/1
  Add7/1 -> Product15/2
  Product15/1 -> P_rt/1, [P_rt]
  [P_rt] -> Product16/1
  [ROU_rt] -> Product16/2
  Product16/1 -> Sqrt/1
  Constant12/1 -> Product17/1
  Sqrt/1 -> Product17/2
  Product17/1 -> [W_5t], W_5t/1
  [W_pr1] -> Add8/2
  [W_pr] -> Add8/1
  Add8/1 -> Product18/1
  Constant13/1 -> Product18/2
  Product18/1 -> dW_pr1/dt/1
  dW_pr1/dt/1 -> W_pr1/1, [W_pr1]
  [W_pr1] -> Add9/2
  [W_pr] -> Add9/1
  [T_rt] -> Add10/2
  [T_st] -> Add10/1
  Constant16/1 -> Product19/2
  Constant15/1 -> Product19/1
  [Q_rt] -> Product20/1
  Constant17/1 -> Product20/2
  Constant14/1 -> Product21/1
  Add9/1 -> Product21/2
  Add10/1 -> Product21/3
  Product19/1 -> Add11/1
  Product20/1 -> Add11/2
  Product21/1 -> Product22/1
  Add11/1 -> Product22/2
  Product22/1 -> dQ_rt/dt/1
  dQ_rt/dt/1 -> Q_rt/1, [Q_rt]
  [C_lb] -> Product23/1
  [P] -> Product23/2
  Product23/1 -> W_pr/1, [W_pr]
  Constant19/1 -> Product24/1
  [P] -> Product24/2
  Constant18/1 -> Add12/1
  Product24/1 -> Add12/2
  Add12/1 -> T_st/1, [T_st]
  Constant20/1 -> Product26/1
  Product7/1 -> Product9/2
  Add6/1 -> Product13/1
  Product13/1 -> dH_rt/dt/1
  [P_rt] -> Product25/1
  [ROU_rt] -> Product25/2
  Product25/1 -> Product26/2
  Product26/1 -> T_rt/1, [T_rt]
  Product9/1 -> Product10/2
  Product10/1 -> Add4/1
  Add4/1 -> Add6/2

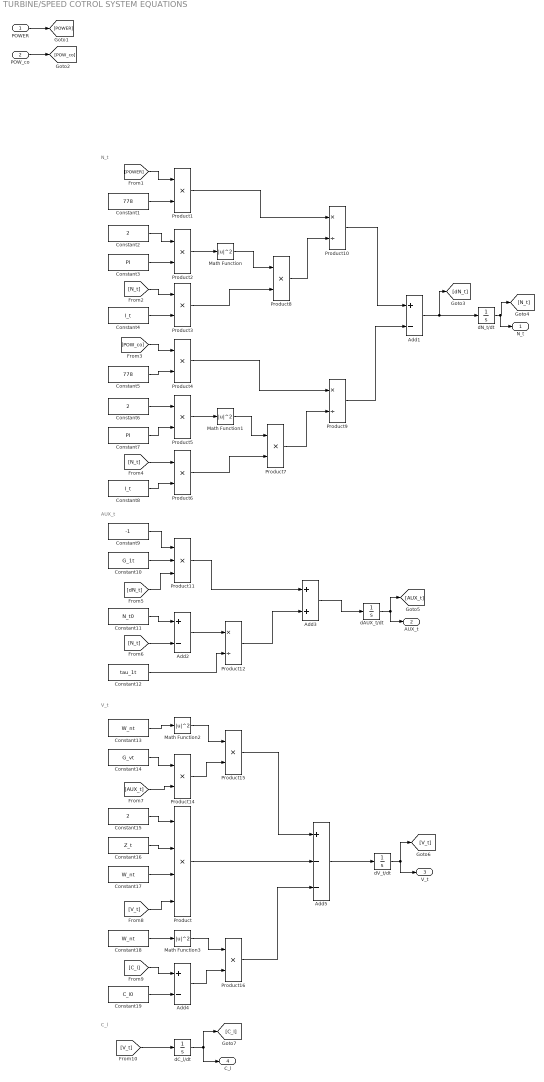
== system TURBINE/SPEED COTROL SYSTEM EQUATIONS ==
  note: C_l
  note: V_t
  note: AUX_t
  note: N_t
  POWER : Inport
  POW_co : Inport  Port=2
  Add1 : Sum  Inputs=+-
  Add2 : Sum  Inputs=+-
  Add3 : Sum
  Add4 : Sum  Inputs=+-
  Add5 : Sum  Inputs=+--
  Constant1 : Constant  Value=778
  Constant10 : Constant  Value=G_1t
  Constant11 : Constant  Value=N_t0
  Constant12 : Constant  Value=tau_1t
  Constant13 : Constant  Value=W_nt
  Constant14 : Constant  Value=G_vt
  Constant15 : Constant  Value=2
  Constant16 : Constant  Value=Z_t
  Constant17 : Constant  Value=W_nt
  Constant18 : Constant  Value=W_nt
  Constant19 : Constant  Value=C_l0
  Constant2 : Constant  Value=2
  Constant3 : Constant  Value=PI
  Constant4 : Constant  Value=I_t
  Constant5 : Constant  Value=778
  Constant6 : Constant  Value=2
  Constant7 : Constant  Value=PI
  Constant8 : Constant  Value=I_t
  Constant9 : Constant  Value=-1
  Math Function{,1..3} (4 alike) : Math  Operator=magnitude^2  SaturateOnIntegerOverflow=on
  Product : Product  Inputs=4
  Product{1..8,14..16} (11 alike) : Product
  Product10 : Product  Inputs=*/
  Product11 : Product  Inputs=3
  Product12 : Product  Inputs=*/
  Product9 : Product  Inputs=*/
  dAUX_t/dt : Integrator
  dC_l/dt : Integrator  InitialCondition=1.2195
  dN_t/dt : Integrator  InitialCondition=60
  dV_t/dt : Integrator
  N_t : Outport
  AUX_t : Outport  Port=2
  V_t : Outport  Port=3
  C_l : Outport  Port=4
  wires:
  POWER/1 -> [POWER]
  POW_co/1 -> [POW_co]
  Constant1/1 -> Product1/2
  [POWER] -> Product1/1
  Constant2/1 -> Product2/1
  Constant3/1 -> Product2/2
  Constant4/1 -> Product3/2
  [N_t] -> Product3/1
  [POW_co] -> Product4/1
  Constant5/1 -> Product4/2
  Constant6/1 -> Product5/1
  Constant7/1 -> Product5/2
  [N_t] -> Product6/1
  Constant8/1 -> Product6/2
  Product2/1 -> Math Function/1
  Product5/1 -> Math Function1/1
  Math Function1/1 -> Product7/1
  Product6/1 -> Product7/2
  Math Function/1 -> Product8/1
  Product3/1 -> Product8/2
  Product4/1 -> Product9/1
  Product7/1 -> Product9/2
  Product8/1 -> Product10/2
  Product1/1 -> Product10/1
  Product10/1 -> Add1/1
  Product9/1 -> Add1/2
  Add1/1 -> [dN_t], dN_t/dt/1
  dN_t/dt/1 -> N_t/1, [N_t]
  Constant9/1 -> Product11/1
  Constant10/1 -> Product11/2
  [dN_t] -> Product11/3
  [N_t] -> Add2/2
  Constant11/1 -> Add2/1
  Product11/1 -> Add3/1
  Constant12/1 -> Product12/2
  dAUX_t/dt/1 -> AUX_t/1, [AUX_t]
  Constant13/1 -> Math Function2/1
  Constant18/1 -> Math Function3/1
  [C_l] -> Add4/1
  Constant19/1 -> Add4/2
  Constant15/1 -> Product/1
  Constant16/1 -> Product/2
  Constant17/1 -> Product/3
  [V_t] -> Product/4
  [AUX_t] -> Product14/2
  Constant14/1 -> Product14/1
  Math Function2/1 -> Product15/1
  Product14/1 -> Product15/2
  Math Function3/1 -> Product16/1
  Add4/1 -> Product16/2
  Product15/1 -> Add5/1
  Product/1 -> Add5/2
  Product16/1 -> Add5/3
  Add5/1 -> dV_t/dt/1
  dV_t/dt/1 -> V_t/1, [V_t]
  [V_t] -> dC_l/dt/1
  dC_l/dt/1 -> C_l/1, [C_l]
  Add2/1 -> Product12/1
  Product12/1 -> Add3/2
  Add3/1 -> dAUX_t/dt/1

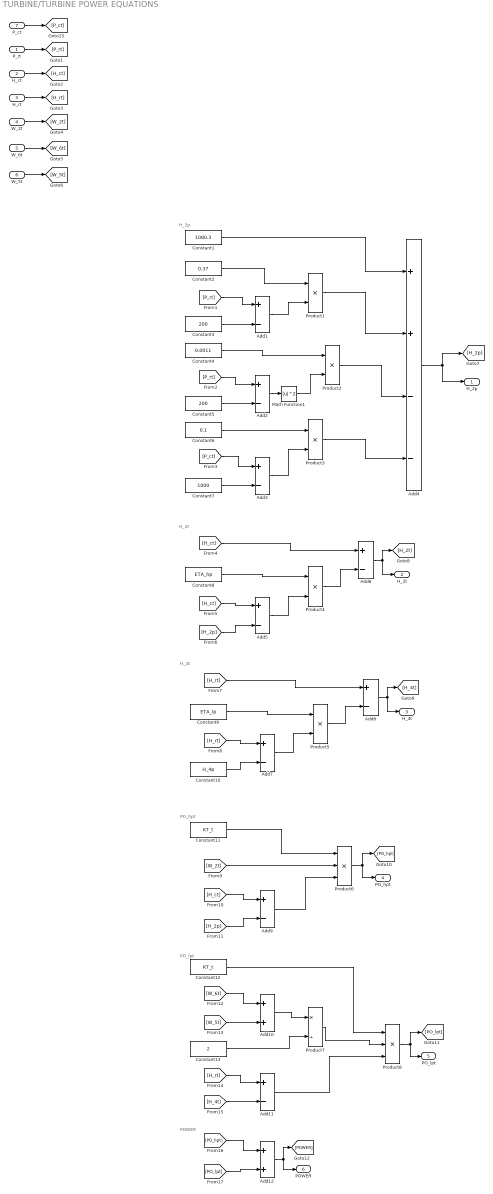
== system TURBINE/TURBINE POWER EQUATIONS ==
  note: POWER
  note: PO_lpt
  note: PO_hpt
  note: H_4t
  note: H_2t
  note: H_2p
  P_rt : Inport
  H_ct : Inport  Port=2
  H_rt : Inport  Port=3
  W_2t : Inport  Port=4
  W_6t : Inport  Port=5
  W_5t : Inport  Port=6
  P_ct : Inport  Port=7
  Add{1..3,5..9,11} (9 alike) : Sum  Inputs=+-
  Add10 : Sum
  Add12 : Sum
  Add4 : Sum  Inputs=++--
  Constant1 : Constant  Value=1080.3
  Constant10 : Constant  Value=H_4p
  Constant11 : Constant  Value=KT_t
  Constant12 : Constant  Value=KT_t
  Constant13 : Constant  Value=2
  Constant2 : Constant  Value=0.37
  Constant3 : Constant  Value=200
  Constant4 : Constant  Value=0.0011
  Constant5 : Constant  Value=200
  Constant6 : Constant  Value=0.1
  Constant7 : Constant  Value=1000
  Constant8 : Constant  Value=ETA_hp
  Constant9 : Constant  Value=ETA_lp
  Math Function1 : Math  Operator=magnitude^2  SaturateOnIntegerOverflow=on
  Product{1..5} (5 alike) : Product
  Product6 : Product  Inputs=3
  Product7 : Product  Inputs=*/
  Product8 : Product  Inputs=3
  H_2p : Outport
  H_2t : Outport  Port=2
  H_4t : Outport  Port=3
  PO_hpt : Outport  Port=4
  PO_lpt : Outport  Port=5
  POWER : Outport  Port=6
  wires:
  P_rt/1 -> [P_rt]
  H_ct/1 -> [H_ct]
  H_rt/1 -> [H_rt]
  W_2t/1 -> [W_2t]
  W_6t/1 -> [W_6t]
  W_5t/1 -> [W_5t]
  P_ct/1 -> [P_ct]
  [P_rt] -> Add1/1
  Constant3/1 -> Add1/2
  Constant2/1 -> Product1/1
  Add1/1 -> Product1/2
  Constant5/1 -> Add2/2
  [P_rt] -> Add2/1
  Constant4/1 -> Product2/1
  Constant7/1 -> Add3/2
  [P_ct] -> Add3/1
  Constant6/1 -> Product3/1
  Add3/1 -> Product3/2
  Constant1/1 -> Add4/1
  Product1/1 -> Add4/2
  Product2/1 -> Add4/3
  Product3/1 -> Add4/4
  Add4/1 -> H_2p/1, [H_2p]
  [H_2p] -> Add5/2
  [H_ct] -> Add5/1
  Constant8/1 -> Product4/1
  Add5/1 -> Product4/2
  [H_ct] -> Add6/1
  Product4/1 -> Add6/2
  Constant10/1 -> Add7/2
  [H_rt] -> Add7/1
  Constant9/1 -> Product5/1
  Add7/1 -> Product5/2
  [H_rt] -> Add8/1
  Product5/1 -> Add8/2
  Add8/1 -> [H_4t], H_4t/1
  Add6/1 -> H_2t/1, [H_2t]
  [H_ct] -> Add9/1
  [H_2p] -> Add9/2
  Constant11/1 -> Product6/1
  [W_2t] -> Product6/2
  Add9/1 -> Product6/3
  Product6/1 -> [PO_hpt], PO_hpt/1
  [W_6t] -> Add10/1
  [W_5t] -> Add10/2
  Add10/1 -> Product7/1
  Constant13/1 -> Product7/2
  [H_rt] -> Add11/1
  [H_4t] -> Add11/2
  Constant12/1 -> Product8/1
  Product7/1 -> Product8/2
  Add11/1 -> Product8/3
  Product8/1 -> PO_lpt/1, [PO_lpt]
  [PO_hpt] -> Add12/1
  [PO_lpt] -> Add12/2
  Add12/1 -> POWER/1, [POWER]
  Add2/1 -> Math Function1/1
  Math Function1/1 -> Product2/2
